simulink library "EnergyMeter_HC"  (Simulink 7.6)
settings: Solver=ode45  StartTime=0.0  StopTime=10.0  RelTol=1e-3
settings Model: Creator=lena.frank  LastModifiedBy=awohlfei

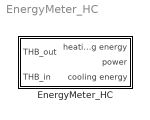
== system EnergyMeter_HC ==
  EnergyMeter_HC : Subsystem
      mask Type: energy meter Heating/Cooling
      mask Description:
      | Calculates the power and energy of a fluid flow between inlet and outlet of components.
      | Positive power is integrated to the heating energy, negative power is integrated to the cooling energy.
      mask Help: eval('htmlhelp (''chap_4_2e.htm#energy_meter'')');

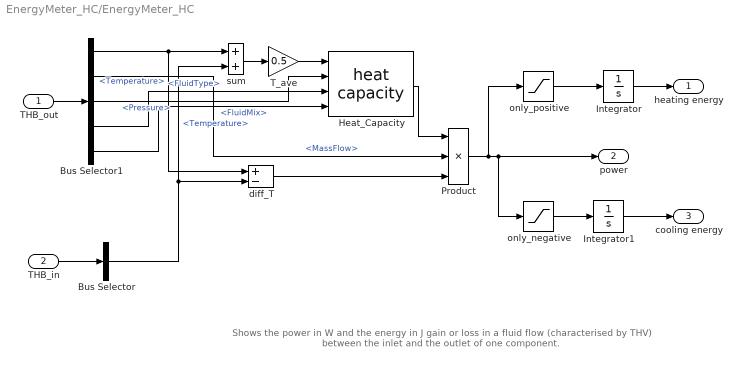
== system EnergyMeter_HC/EnergyMeter_HC ==
  note: Shows the power in W and the energy in J gain or loss
      | in a fluid flow (characterised by THV) between the
      | inlet and the outlet of one component.
  THB_out : Inport
  THB_in : Inport  Port=2
  Bus Selector : BusSelector  OutputSignals=Temperature
  Bus Selector1 : BusSelector  OutputSignals=Temperature,MassFlow,Pressure,FluidType,FluidMix
  Heat_Capacity : Reference  SystemSampleTime=-1
  Integrator : Integrator  UpperSaturationLimit=1  LowerSaturationLimit=0
  Integrator1 : Integrator  UpperSaturationLimit=1  LowerSaturationLimit=0
  Product : Product  Inputs=***  SaturateOnIntegerOverflow=on  RndMeth=Zero  InputSameDT=on  OutDataTypeStr=Inherit: Same as first input
  T_ave : Gain  Gain=0.5  SaturateOnIntegerOverflow=on  OutDataTypeStr=Inherit: Same as input  ParamDataTypeStr=Inherit: Same as input
  diff_T : Sum  Inputs=+-  SaturateOnIntegerOverflow=on  InputSameDT=on  OutDataTypeStr=Inherit: Same as first input
  only_negative : Saturate  UpperLimit=0  LowerLimit=-inf
  only_positive : Saturate  UpperLimit=inf  LowerLimit=0
  sum : Sum  SaturateOnIntegerOverflow=on  InputSameDT=on  OutDataTypeStr=Inherit: Same as first input
  heating energy : Outport  InitialOutput=0
  power : Outport  Port=2  InitialOutput=0
  cooling energy : Outport  Port=3  InitialOutput=0
  wires:
  only_positive/1 -> Integrator/1
  only_negative/1 -> Integrator1/1
  Product/1 -> only_positive/1, only_negative/1, power/1
  Integrator1/1 -> cooling energy/1
  Bus Selector1/3 -> Heat_Capacity/2  "<Pressure>"
  T_ave/1 -> Heat_Capacity/1
  sum/1 -> T_ave/1
  Bus Selector/1 -> sum/2, diff_T/2  "<Temperature>"
  diff_T/1 -> Product/3
  Bus Selector1/2 -> Product/2  "<MassFlow>"
  Integrator/1 -> heating energy/1
  Heat_Capacity/1 -> Product/1
  Bus Selector1/5 -> Heat_Capacity/4  "<FluidMix>"
  Bus Selector1/4 -> Heat_Capacity/3  "<FluidType>"
  Bus Selector1/1 -> sum/1, diff_T/1  "<Temperature>"
  THB_out/1 -> Bus Selector1/1
  THB_in/1 -> Bus Selector/1
